simulink model "MobileManipulatorSlave"  (R2016a)
settings: Solver=FixedStepDiscrete  SolverMode=SingleTasking  StartTime=0.0  StopTime=inf  FixedStep=.001  RelTol=1e-3
undefined symbols (not defined in the file): DiscIntNeverNeededParam, transl
libraries: simulink x18, dspfactors x1, LibrarySimulinkSAS x1, aerolibanimutils x1, dspnetwork x1
settings Model: xpc_rtwmakecfg_data=_jpeg_  Creator=DSANTIAGO  LastModifiedBy=INAUT
settings DataIOCC: LimitDataPoints=on  SaveFormat=Array
settings OptimizationCC: BlockReduction=off  BooleanDataType=off
settings DebuggingCC: SaveWithParameterizedLinksMsg=none  UnderspecifiedInitializationDetection=Classic  MergeDetectMultiDrivingBlocksExec=none  SignalResolutionControl=TryResolveAllWithWarning  InvalidFcnCallConnMsg=warning  FcnCallInpInsideContextMsg=EnableAllAsWarning
settings HardwareCC: ProdBitPerPointer=32  ProdLargestAtomicFloat=None  ProdIntDivRoundTo=Undefined  ProdEndianess=Unspecified  ProdWordSize=32  ProdHWDeviceType=32-bit Generic  TargetUnknown=on
settings ModelReferenceCC: PropagateSignalLabelsOutOfModel=off
settings ConfigComp: CovSFcnEnable=off

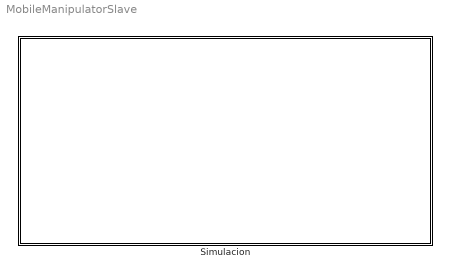
== system MobileManipulatorSlave ==
  Simulacion : Subsystem  mask{sel=1, offSet=[1.5e-1 0 0.1]', h1=.01, h2=.01, kgmb=diag([8 10]), kgms=diag([4 4 4]), kms=10, kmb=5, ksb=1}
      mask prompts: sel "Control (s/m)"; h1 "Delay1"; h2 "Delay2"

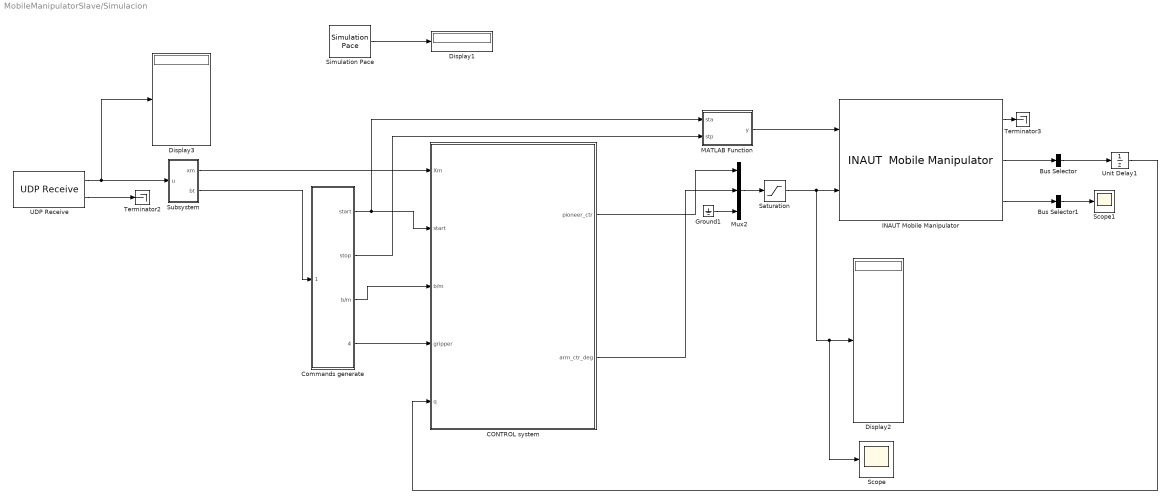
== system MobileManipulatorSlave/Simulacion ==
  Bus Selector : BusSelector  OutputSignals=q_{arm}  OutputAsBus=on
  Bus Selector1 : BusSelector  OutputSignals=base Info.current rigth motor?,base Info.current left motor?  OutputAsBus=on
  CONTROL system : Subsystem
  Commands generate : Subsystem
  Display1 : Display
  Display2 : Display
  Display3 : Display
  Ground1 : Ground
  INAUT Mobile Manipulator : LibrarySimulinkSAS/INAUT  Mobile Manipulator  IdB=3  IdM=1  IdL=0  ts=-1
  MATLAB Function : MATLAB Function  TreatAsAtomicUnit=on
  Mux2 : Mux  Inputs=3
  Saturation : Saturate  UpperLimit=2000  LowerLimit=-2000
  Scope : Scope
  Scope1 : Scope
  Simulation Pace : aerolibanimutils/Simulation Pace  SimulationPace=1  SleepMode=MATLAB Thread  OutputPaceError=on  SampleTime=-1
  Subsystem : Subsystem
  Terminator2 : Terminator
  Terminator3 : Terminator
  UDP Receive : dspnetwork/UDP Receive  localURL='0.0.0.0'  localPort=24102  remoteURL='192.168.1.103'  remotePort=-1  recvBufferSize=1024  dims=7  signalDatatype=double  isVarSize=off  showBlockingTime=off  blockingTime=0  sampletime=-1  blockPlatform=[]
  Unit Delay1 : UnitDelay  SampleTime=-1
  wires:
  Subsystem/1(xm) -> CONTROL system/1(Xm)
  Unit Delay1/1 -> CONTROL system/5(q)
  Subsystem/2(bt) -> Commands generate/1(butons)
  Commands generate/1(start) -> MATLAB Function/1(sta), CONTROL system/2(start)
  CONTROL system/2(arm_ctr_deg) -> Mux2/2
  Mux2/1 -> Saturation/1
  INAUT Mobile Manipulator/2 -> Bus Selector/1
  INAUT Mobile Manipulator/3 -> Bus Selector1/1
  INAUT Mobile Manipulator/1 -> Terminator3/1
  Bus Selector/1 -> Unit Delay1/1
  CONTROL system/1(pioneer_ctr) -> Mux2/1
  Ground1/1 -> Mux2/3
  Simulation Pace/1 -> Display1/1
  Commands generate/3(b/m) -> CONTROL system/3(b/m)
  Commands generate/4(griper) -> CONTROL system/4(gripper)
  UDP Receive/1 -> Subsystem/1(u), Display3/1
  UDP Receive/2 -> Terminator2/1
  Saturation/1 -> Scope/1, Display2/1, INAUT Mobile Manipulator/2
  Bus Selector1/1 -> Scope1/1
  MATLAB Function/1(y) -> INAUT Mobile Manipulator/1
  Commands generate/2(stop) -> MATLAB Function/2(stp)

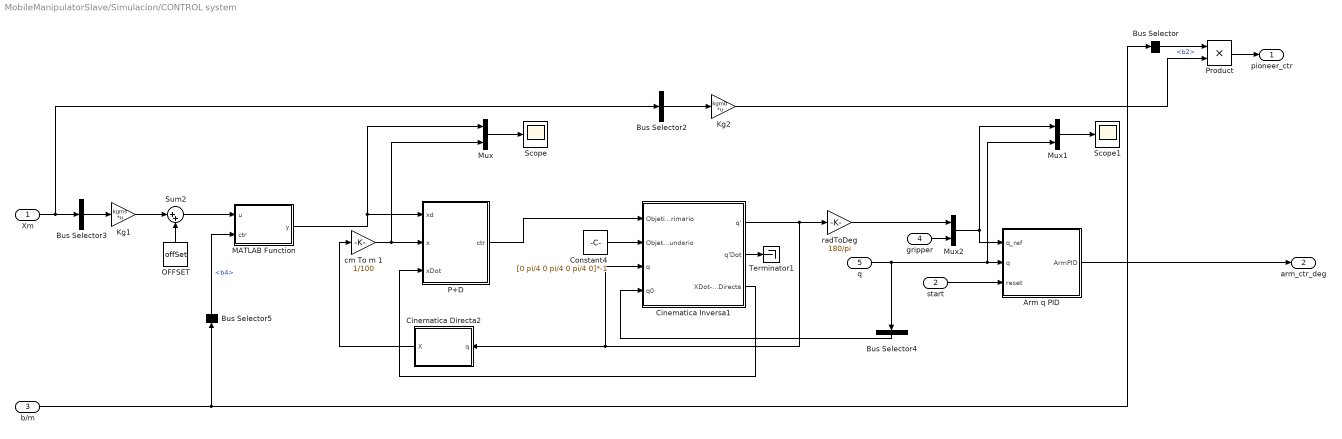
== system MobileManipulatorSlave/Simulacion/CONTROL system ==
  Xm : Inport
  start : Inport  Port=2
  b/m : Inport  Port=3
  gripper : Inport  Port=4
  q : Inport  Port=5
  Arm q PID : Subsystem
  Bus Selector : BusSelector  OutputSignals=b2
  Bus Selector2 : BusSelector  OutputSignals=x,y  OutputAsBus=on
  Bus Selector3 : BusSelector  OutputSignals=x,y,z  OutputAsBus=on
  Bus Selector4 : BusSelector  OutputSignals=q1,q2,q3,q4,q5,q6,q7  OutputAsBus=on
  Bus Selector5 : BusSelector  OutputSignals=b4
  Cinematica Directa2 : Subsystem
  Cinematica Inversa1 : Subsystem
  Constant4 : Constant  Value=[0 pi/4 0 pi/4 0 pi/4 0]*-1
  Kg1 : Gain  Gain=kgms  Multiplication=Matrix(K*u)
  Kg2 : Gain  Gain=kgmb  Multiplication=Matrix(K*u)
  MATLAB Function : MATLAB Function  TreatAsAtomicUnit=on
  Mux : Mux  Inputs=2
  Mux1 : Mux  Inputs=2
  Mux2 : Mux  Inputs=2
  OFFSET : Constant  Value=offSet
  P+D : Subsystem
  Product : Product
  Scope : Scope
  Scope1 : Scope
  Sum2 : Sum  Inputs=|++
  Terminator1 : Terminator
  cm To m 1 : Gain  Gain=1/100
  radToDeg : Gain  Gain=180/pi
  pioneer_ctr : Outport
  arm_ctr_deg : Outport  Port=2
  wires:
  Xm/1 -> Bus Selector3/1, Bus Selector2/1
  Bus Selector2/1 -> Kg2/1
  Cinematica Inversa1/1(q') -> Cinematica Inversa1/3(q), Cinematica Directa2/1(q), radToDeg/1
  OFFSET/1 -> Sum2/2
  Kg1/1 -> Sum2/1
  P+D/1(ctr) -> Cinematica Inversa1/1(Objetivo Primario)
  Cinematica Directa2/1("X ") -> cm To m 1/1
  cm To m 1/1 -> Mux/2, P+D/2(x)
  Constant4/1 -> Cinematica Inversa1/2(Objetivo Secundario)
  gripper/1 -> Mux2/2
  start/1 -> Arm q PID/3(reset)
  b/m/1 -> Bus Selector5/1, Bus Selector/1
  Bus Selector/1 -> Product/1  "<b2>"
  Kg2/1 -> Product/2
  radToDeg/1 -> Mux2/1
  Sum2/1 -> MATLAB Function/1(u)
  Product/1 -> pioneer_ctr/1
  Cinematica Inversa1/2(q'Dot) -> Terminator1/1
  Bus Selector3/1 -> Kg1/1
  Mux/1 -> Scope/1
  Cinematica Inversa1/3(XDot- CinematicaDirecta) -> P+D/3(xDot)
  q/1 -> Bus Selector4/1, Mux1/2, Arm q PID/2(q)
  Mux2/1 -> Mux1/1, Arm q PID/1(q_ref)
  Mux1/1 -> Scope1/1
  Bus Selector4/1 -> Cinematica Inversa1/4(q0)
  MATLAB Function/1(y) -> Mux/1, P+D/1(xd)
  Bus Selector5/1 -> MATLAB Function/2(ctr)  "<b4>"
  Arm q PID/1(ArmPID) -> arm_ctr_deg/1

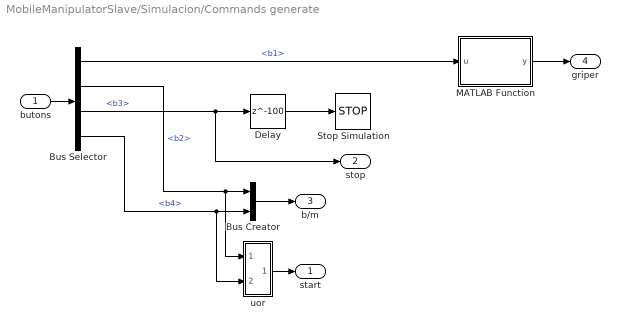
== system MobileManipulatorSlave/Simulacion/Commands generate ==
  butons : Inport
  Bus Creator : BusCreator  Inputs=2
  Bus Selector : BusSelector  OutputSignals=b1,b2,b3,b4
  Delay : Delay  DelayLength=100
  MATLAB Function : MATLAB Function  TreatAsAtomicUnit=on
  Stop Simulation : Stop
  uor : Subsystem
  start : Outport
  stop : Outport  Port=2
  b/m : Outport  Port=3
  griper : Outport  Port=4
  wires:
  Bus Selector/2 -> uor/1(u1), Bus Creator/1  "<b2>"
  Bus Selector/3 -> stop/1, Delay/1  "<b3>"
  Delay/1 -> Stop Simulation/1
  Bus Creator/1 -> b/m/1
  Bus Selector/4 -> uor/2(u2), Bus Creator/2  "<b4>"
  Bus Selector/1 -> MATLAB Function/1(u)  "<b1>"
  butons/1 -> Bus Selector/1
  uor/1(y) -> start/1
  MATLAB Function/1(y) -> griper/1

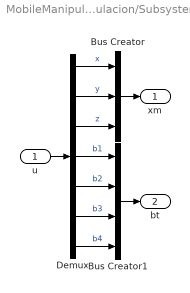
== system MobileManipulatorSlave/Simulacion/Subsystem ==
  u : Inport
  Bus Creator : BusCreator  Inputs=3
  Bus Creator1 : BusCreator  Inputs=4
  Demux : Demux  Outputs=7
  xm : Outport
  bt : Outport  Port=2
  wires:
  Demux/2 -> Bus Creator/2  "y"
  Demux/3 -> Bus Creator/3  "z"
  Demux/5 -> Bus Creator1/2  "b2"
  Demux/1 -> Bus Creator/1  "x"
  Demux/6 -> Bus Creator1/3  "b3"
  Demux/4 -> Bus Creator1/1  "b1"
  Demux/7 -> Bus Creator1/4  "b4"
  Bus Creator1/1 -> bt/1
  u/1 -> Demux/1
  Bus Creator/1 -> xm/1

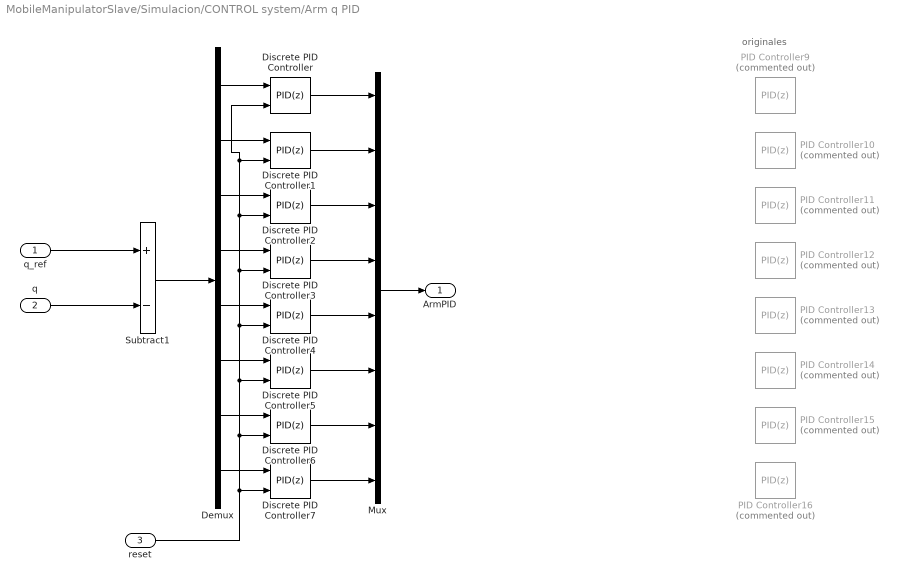
== system MobileManipulatorSlave/Simulacion/CONTROL system/Arm q PID ==
  note: originales
  q_ref : Inport
  q : Inport  Port=2
  reset : Inport  Port=3
  Demux : Demux  Outputs=8
  Discrete PID Controller : simulink/Continuous/PID Controller  Controller=PID  TimeDomain=Discrete-time  SampleTime=-1  IntegratorMethod=Forward Euler  FilterMethod=Forward Euler  Form=Parallel  UseFilter=on  ControllerParametersSource=internal  P=125  I=40  D=0.01  N=100  InitialConditionSource=internal  InitialConditionForIntegrator=0  InitialConditionForFilter=0  ExternalReset=level  LimitOutput=on  UpperSaturationLimit=4095  LowerSaturationLimit=-4095  LinearizeAsGain=on  AntiWindupMode=clamping  Kb=1  TrackingMode=off  Kt=1  PParamMin=[]  PParamMax=[]  IParamMin=[]  IParamMax=[]  DParamMin=[]  DParamMax=[]  NParamMin=[]  NParamMax=[]  KbParamMin=[]  KbParamMax=[]  KtParamMin=[]  KtParamMax=[]  POutMin=[]  POutMax=[]  IOutMin=[]  IOutMax=[]  DOutMin=[]  DOutMax=[]  NOutMin=[]  NOutMax=[]  KbOutMin=[]  KbOutMax=[]  KtOutMin=[]  KtOutMax=[]  IntegratorOutMin=[]  IntegratorOutMax=[]  FilterOutMin=[]  FilterOutMax=[]  SumOutMin=[]  SumOutMax=[]  SumI1OutMin=[]  SumI1OutMax=[]  SumI2OutMin=[]  SumI2OutMax=[]  SumI3OutMin=[]  SumI3OutMax=[]  SumDOutMin=[]  SumDOutMax=[]  SaturationOutMin=[]  SaturationOutMax=[]  IntegratorContinuousStateAttributes=''  IntegratorStateMustResolveToSignalObject=off  IntegratorRTWStateStorageClass=Auto  FilterContinuousStateAttributes=''  FilterStateMustResolveToSignalObject=off  FilterRTWStateStorageClass=Auto  DifferentiatorICPrevScaledInput=0  DifferentiatorOutMin=[]  DifferentiatorOutMax=[]
  Discrete PID Controller1 : simulink/Continuous/PID Controller  Controller=PID  TimeDomain=Discrete-time  SampleTime=-1  IntegratorMethod=Forward Euler  FilterMethod=Forward Euler  Form=Parallel  UseFilter=on  ControllerParametersSource=internal  P=75  I=100  D=0.01  N=100  InitialConditionSource=internal  InitialConditionForIntegrator=0  InitialConditionForFilter=0  ExternalReset=level  LimitOutput=on  UpperSaturationLimit=4095  LowerSaturationLimit=-4095  LinearizeAsGain=on  AntiWindupMode=clamping  Kb=1  TrackingMode=off  Kt=1  PParamMin=[]  PParamMax=[]  IParamMin=[]  IParamMax=[]  DParamMin=[]  DParamMax=[]  NParamMin=[]  NParamMax=[]  KbParamMin=[]  KbParamMax=[]  KtParamMin=[]  KtParamMax=[]  POutMin=[]  POutMax=[]  IOutMin=[]  IOutMax=[]  DOutMin=[]  DOutMax=[]  NOutMin=[]  NOutMax=[]  KbOutMin=[]  KbOutMax=[]  KtOutMin=[]  KtOutMax=[]  IntegratorOutMin=[]  IntegratorOutMax=[]  FilterOutMin=[]  FilterOutMax=[]  SumOutMin=[]  SumOutMax=[]  SumI1OutMin=[]  SumI1OutMax=[]  SumI2OutMin=[]  SumI2OutMax=[]  SumI3OutMin=[]  SumI3OutMax=[]  SumDOutMin=[]  SumDOutMax=[]  SaturationOutMin=[]  SaturationOutMax=[]  IntegratorContinuousStateAttributes=''  IntegratorStateMustResolveToSignalObject=off  IntegratorRTWStateStorageClass=Auto  FilterContinuousStateAttributes=''  FilterStateMustResolveToSignalObject=off  FilterRTWStateStorageClass=Auto  DifferentiatorICPrevScaledInput=0  DifferentiatorOutMin=[]  DifferentiatorOutMax=[]
  Discrete PID Controller2 : simulink/Continuous/PID Controller  Controller=PID  TimeDomain=Discrete-time  SampleTime=-1  IntegratorMethod=Forward Euler  FilterMethod=Forward Euler  Form=Parallel  UseFilter=on  ControllerParametersSource=internal  P=80  I=45  D=0.01  N=100  InitialConditionSource=internal  InitialConditionForIntegrator=0  InitialConditionForFilter=0  ExternalReset=level  LimitOutput=on  UpperSaturationLimit=4095  LowerSaturationLimit=-4095  LinearizeAsGain=on  AntiWindupMode=clamping  Kb=1  TrackingMode=off  Kt=1  PParamMin=[]  PParamMax=[]  IParamMin=[]  IParamMax=[]  DParamMin=[]  DParamMax=[]  NParamMin=[]  NParamMax=[]  KbParamMin=[]  KbParamMax=[]  KtParamMin=[]  KtParamMax=[]  POutMin=[]  POutMax=[]  IOutMin=[]  IOutMax=[]  DOutMin=[]  DOutMax=[]  NOutMin=[]  NOutMax=[]  KbOutMin=[]  KbOutMax=[]  KtOutMin=[]  KtOutMax=[]  IntegratorOutMin=[]  IntegratorOutMax=[]  FilterOutMin=[]  FilterOutMax=[]  SumOutMin=[]  SumOutMax=[]  SumI1OutMin=[]  SumI1OutMax=[]  SumI2OutMin=[]  SumI2OutMax=[]  SumI3OutMin=[]  SumI3OutMax=[]  SumDOutMin=[]  SumDOutMax=[]  SaturationOutMin=[]  SaturationOutMax=[]  IntegratorContinuousStateAttributes=''  IntegratorStateMustResolveToSignalObject=off  IntegratorRTWStateStorageClass=Auto  FilterContinuousStateAttributes=''  FilterStateMustResolveToSignalObject=off  FilterRTWStateStorageClass=Auto  DifferentiatorICPrevScaledInput=0  DifferentiatorOutMin=[]  DifferentiatorOutMax=[]
  Discrete PID Controller{3..7} (5 alike) : simulink/Continuous/PID Controller  Controller=PID  TimeDomain=Discrete-time  SampleTime=-1  IntegratorMethod=Forward Euler  FilterMethod=Forward Euler  Form=Parallel  UseFilter=on  ControllerParametersSource=internal  P=75  I=40  D=0.01  N=100  InitialConditionSource=internal  InitialConditionForIntegrator=0  InitialConditionForFilter=0  ExternalReset=level  LimitOutput=on  UpperSaturationLimit=4095  LowerSaturationLimit=-4095  LinearizeAsGain=on  AntiWindupMode=clamping  Kb=1  TrackingMode=off  Kt=1  PParamMin=[]  PParamMax=[]  IParamMin=[]  IParamMax=[]  DParamMin=[]  DParamMax=[]  NParamMin=[]  NParamMax=[]  KbParamMin=[]  KbParamMax=[]  KtParamMin=[]  KtParamMax=[]  POutMin=[]  POutMax=[]  IOutMin=[]  IOutMax=[]  DOutMin=[]  DOutMax=[]  NOutMin=[]  NOutMax=[]  KbOutMin=[]  KbOutMax=[]  KtOutMin=[]  KtOutMax=[]  IntegratorOutMin=[]  IntegratorOutMax=[]  FilterOutMin=[]  FilterOutMax=[]  SumOutMin=[]  SumOutMax=[]  SumI1OutMin=[]  SumI1OutMax=[]  SumI2OutMin=[]  SumI2OutMax=[]  SumI3OutMin=[]  SumI3OutMax=[]  SumDOutMin=[]  SumDOutMax=[]  SaturationOutMin=[]  SaturationOutMax=[]  IntegratorContinuousStateAttributes=''  IntegratorStateMustResolveToSignalObject=off  IntegratorRTWStateStorageClass=Auto  FilterContinuousStateAttributes=''  FilterStateMustResolveToSignalObject=off  FilterRTWStateStorageClass=Auto  DifferentiatorICPrevScaledInput=0  DifferentiatorOutMin=[]  DifferentiatorOutMax=[]
  Mux : Mux  Inputs=8
  PID Controller10 : simulink/Continuous/PID Controller  Commented=on  Controller=PID  TimeDomain=Discrete-time  SampleTime=-1  IntegratorMethod=Forward Euler  FilterMethod=Forward Euler  Form=Parallel  UseFilter=on  ControllerParametersSource=internal  P=75  I=100  D=0.01  N=100  InitialConditionSource=internal  InitialConditionForIntegrator=0  InitialConditionForFilter=0  ExternalReset=rising  LimitOutput=on  UpperSaturationLimit=4095  LowerSaturationLimit=-4095  LinearizeAsGain=on  AntiWindupMode=clamping  Kb=1  TrackingMode=off  Kt=1  PParamMin=[]  PParamMax=[]  PParamDataTypeStr=single  IParamMin=[]  IParamMax=[]  IParamDataTypeStr=single  DParamMin=[]  DParamMax=[]  DParamDataTypeStr=single  NParamMin=[]  NParamMax=[]  NParamDataTypeStr=single  KbParamMin=[]  KbParamMax=[]  KtParamMin=[]  KtParamMax=[]  POutMin=[]  POutMax=[]  POutDataTypeStr=single  PGainOutDataTypeStr=single  PProdOutDataTypeStr=single  IOutMin=[]  IOutMax=[]  IOutDataTypeStr=single  IGainOutDataTypeStr=single  IProdOutDataTypeStr=single  DOutMin=[]  DOutMax=[]  DOutDataTypeStr=single  DGainOutDataTypeStr=single  DProdOutDataTypeStr=single  NOutMin=[]  NOutMax=[]  NOutDataTypeStr=single  NGainOutDataTypeStr=single  NProdOutDataTypeStr=single  KbOutMin=[]  KbOutMax=[]  KtOutMin=[]  KtOutMax=[]  IntegratorOutMin=[]  IntegratorOutMax=[]  IntegratorOutDataTypeStr=single  FilterOutMin=[]  FilterOutMax=[]  FilterOutDataTypeStr=single  SumOutMin=[]  SumOutMax=[]  SumOutDataTypeStr=single  SumI1OutMin=[]  SumI1OutMax=[]  SumI2OutMin=[]  SumI2OutMax=[]  SumI3OutMin=[]  SumI3OutMax=[]  SumDOutMin=[]  SumDOutMax=[]  SumDOutDataTypeStr=single  SumAccumDataTypeStr=single  SumDAccumDataTypeStr=single  SaturationOutMin=[]  SaturationOutMax=[]  SaturationOutDataTypeStr=single  IntegratorContinuousStateAttributes=''  IntegratorStateMustResolveToSignalObject=off  IntegratorRTWStateStorageClass=Auto  FilterContinuousStateAttributes=''  FilterStateMustResolveToSignalObject=off  FilterRTWStateStorageClass=Auto  DifferentiatorICPrevScaledInput=0  DifferentiatorOutMin=[]  DifferentiatorOutMax=[]
  PID Controller11 : simulink/Continuous/PID Controller  Commented=on  Controller=PID  TimeDomain=Discrete-time  SampleTime=-1  IntegratorMethod=Forward Euler  FilterMethod=Forward Euler  Form=Parallel  UseFilter=on  ControllerParametersSource=internal  P=80  I=45  D=0.01  N=100  InitialConditionSource=internal  InitialConditionForIntegrator=0  InitialConditionForFilter=0  ExternalReset=rising  LimitOutput=on  UpperSaturationLimit=4095  LowerSaturationLimit=-4095  LinearizeAsGain=on  AntiWindupMode=clamping  Kb=1  TrackingMode=off  Kt=1  PParamMin=[]  PParamMax=[]  PParamDataTypeStr=single  IParamMin=[]  IParamMax=[]  IParamDataTypeStr=single  DParamMin=[]  DParamMax=[]  DParamDataTypeStr=single  NParamMin=[]  NParamMax=[]  NParamDataTypeStr=single  KbParamMin=[]  KbParamMax=[]  KtParamMin=[]  KtParamMax=[]  POutMin=[]  POutMax=[]  POutDataTypeStr=single  PGainOutDataTypeStr=single  PProdOutDataTypeStr=single  IOutMin=[]  IOutMax=[]  IOutDataTypeStr=single  IGainOutDataTypeStr=single  IProdOutDataTypeStr=single  DOutMin=[]  DOutMax=[]  DOutDataTypeStr=single  DGainOutDataTypeStr=single  DProdOutDataTypeStr=single  NOutMin=[]  NOutMax=[]  NOutDataTypeStr=single  NGainOutDataTypeStr=single  NProdOutDataTypeStr=single  KbOutMin=[]  KbOutMax=[]  KtOutMin=[]  KtOutMax=[]  IntegratorOutMin=[]  IntegratorOutMax=[]  IntegratorOutDataTypeStr=single  FilterOutMin=[]  FilterOutMax=[]  FilterOutDataTypeStr=single  SumOutMin=[]  SumOutMax=[]  SumOutDataTypeStr=single  SumI1OutMin=[]  SumI1OutMax=[]  SumI2OutMin=[]  SumI2OutMax=[]  SumI3OutMin=[]  SumI3OutMax=[]  SumDOutMin=[]  SumDOutMax=[]  SumDOutDataTypeStr=single  SumAccumDataTypeStr=single  SumDAccumDataTypeStr=single  SaturationOutMin=[]  SaturationOutMax=[]  SaturationOutDataTypeStr=single  IntegratorContinuousStateAttributes=''  IntegratorStateMustResolveToSignalObject=off  IntegratorRTWStateStorageClass=Auto  FilterContinuousStateAttributes=''  FilterStateMustResolveToSignalObject=off  FilterRTWStateStorageClass=Auto  DifferentiatorICPrevScaledInput=0  DifferentiatorOutMin=[]  DifferentiatorOutMax=[]
  PID Controller{12..16} (5 alike) : simulink/Continuous/PID Controller  Commented=on  Controller=PID  TimeDomain=Discrete-time  SampleTime=-1  IntegratorMethod=Forward Euler  FilterMethod=Forward Euler  Form=Parallel  UseFilter=on  ControllerParametersSource=internal  P=75  I=40  D=0.01  N=100  InitialConditionSource=internal  InitialConditionForIntegrator=0  InitialConditionForFilter=0  ExternalReset=rising  LimitOutput=on  UpperSaturationLimit=4095  LowerSaturationLimit=-4095  LinearizeAsGain=on  AntiWindupMode=clamping  Kb=1  TrackingMode=off  Kt=1  PParamMin=[]  PParamMax=[]  PParamDataTypeStr=single  IParamMin=[]  IParamMax=[]  IParamDataTypeStr=single  DParamMin=[]  DParamMax=[]  DParamDataTypeStr=single  NParamMin=[]  NParamMax=[]  NParamDataTypeStr=single  KbParamMin=[]  KbParamMax=[]  KtParamMin=[]  KtParamMax=[]  POutMin=[]  POutMax=[]  POutDataTypeStr=single  PGainOutDataTypeStr=single  PProdOutDataTypeStr=single  IOutMin=[]  IOutMax=[]  IOutDataTypeStr=single  IGainOutDataTypeStr=single  IProdOutDataTypeStr=single  DOutMin=[]  DOutMax=[]  DOutDataTypeStr=single  DGainOutDataTypeStr=single  DProdOutDataTypeStr=single  NOutMin=[]  NOutMax=[]  NOutDataTypeStr=single  NGainOutDataTypeStr=single  NProdOutDataTypeStr=single  KbOutMin=[]  KbOutMax=[]  KtOutMin=[]  KtOutMax=[]  IntegratorOutMin=[]  IntegratorOutMax=[]  IntegratorOutDataTypeStr=single  FilterOutMin=[]  FilterOutMax=[]  FilterOutDataTypeStr=single  SumOutMin=[]  SumOutMax=[]  SumOutDataTypeStr=single  SumI1OutMin=[]  SumI1OutMax=[]  SumI2OutMin=[]  SumI2OutMax=[]  SumI3OutMin=[]  SumI3OutMax=[]  SumDOutMin=[]  SumDOutMax=[]  SumDOutDataTypeStr=single  SumAccumDataTypeStr=single  SumDAccumDataTypeStr=single  SaturationOutMin=[]  SaturationOutMax=[]  SaturationOutDataTypeStr=single  IntegratorContinuousStateAttributes=''  IntegratorStateMustResolveToSignalObject=off  IntegratorRTWStateStorageClass=Auto  FilterContinuousStateAttributes=''  FilterStateMustResolveToSignalObject=off  FilterRTWStateStorageClass=Auto  DifferentiatorICPrevScaledInput=0  DifferentiatorOutMin=[]  DifferentiatorOutMax=[]
  PID Controller9 : simulink/Continuous/PID Controller  Commented=on  Controller=PID  TimeDomain=Discrete-time  SampleTime=-1  IntegratorMethod=Forward Euler  FilterMethod=Forward Euler  Form=Parallel  UseFilter=on  ControllerParametersSource=internal  P=125  I=40  D=0.01  N=100  InitialConditionSource=internal  InitialConditionForIntegrator=0  InitialConditionForFilter=0  ExternalReset=level  LimitOutput=on  UpperSaturationLimit=4095  LowerSaturationLimit=-4095  LinearizeAsGain=on  AntiWindupMode=clamping  Kb=1  TrackingMode=off  Kt=1  PParamMin=[]  PParamMax=[]  PParamDataTypeStr=single  IParamMin=[]  IParamMax=[]  IParamDataTypeStr=single  DParamMin=[]  DParamMax=[]  DParamDataTypeStr=single  NParamMin=[]  NParamMax=[]  NParamDataTypeStr=single  KbParamMin=[]  KbParamMax=[]  KtParamMin=[]  KtParamMax=[]  POutMin=[]  POutMax=[]  POutDataTypeStr=single  PGainOutDataTypeStr=single  PProdOutDataTypeStr=single  IOutMin=[]  IOutMax=[]  IOutDataTypeStr=single  IGainOutDataTypeStr=single  IProdOutDataTypeStr=single  DOutMin=[]  DOutMax=[]  DOutDataTypeStr=single  DGainOutDataTypeStr=single  DProdOutDataTypeStr=single  NOutMin=[]  NOutMax=[]  NOutDataTypeStr=single  NGainOutDataTypeStr=single  NProdOutDataTypeStr=single  KbOutMin=[]  KbOutMax=[]  KtOutMin=[]  KtOutMax=[]  IntegratorOutMin=[]  IntegratorOutMax=[]  IntegratorOutDataTypeStr=single  FilterOutMin=[]  FilterOutMax=[]  FilterOutDataTypeStr=single  SumOutMin=[]  SumOutMax=[]  SumOutDataTypeStr=single  SumI1OutMin=[]  SumI1OutMax=[]  SumI2OutMin=[]  SumI2OutMax=[]  SumI3OutMin=[]  SumI3OutMax=[]  SumDOutMin=[]  SumDOutMax=[]  SumDOutDataTypeStr=single  SumAccumDataTypeStr=single  SumDAccumDataTypeStr=single  SaturationOutMin=[]  SaturationOutMax=[]  SaturationOutDataTypeStr=single  IntegratorContinuousStateAttributes=''  IntegratorStateMustResolveToSignalObject=off  IntegratorRTWStateStorageClass=Auto  FilterContinuousStateAttributes=''  FilterStateMustResolveToSignalObject=off  FilterRTWStateStorageClass=Auto  DifferentiatorICPrevScaledInput=0  DifferentiatorOutMin=[]  DifferentiatorOutMax=[]
  Subtract1 : Sum  Inputs=+-
  ArmPID : Outport  PortDimensions=8
  wires:
  q/1 -> Subtract1/2
  q_ref/1 -> Subtract1/1
  Demux/1 -> Discrete PID Controller/1
  Subtract1/1 -> Demux/1
  Demux/6 -> Discrete PID Controller5/1
  Demux/2 -> Discrete PID Controller1/1
  Demux/3 -> Discrete PID Controller2/1
  Demux/4 -> Discrete PID Controller3/1
  Demux/5 -> Discrete PID Controller4/1
  Demux/7 -> Discrete PID Controller6/1
  Demux/8 -> Discrete PID Controller7/1
  Discrete PID Controller7/1 -> Mux/8
  Discrete PID Controller6/1 -> Mux/7
  Discrete PID Controller5/1 -> Mux/6
  Discrete PID Controller4/1 -> Mux/5
  Discrete PID Controller3/1 -> Mux/4
  Discrete PID Controller2/1 -> Mux/3
  Discrete PID Controller1/1 -> Mux/2
  reset/1 -> Discrete PID Controller7/2, Discrete PID Controller6/2, Discrete PID Controller5/2, Discrete PID Controller4/2, Discrete PID Controller3/2, Discrete PID Controller2/2, Discrete PID Controller1/2, Discrete PID Controller/2
  Discrete PID Controller/1 -> Mux/1
  Mux/1 -> ArmPID/1

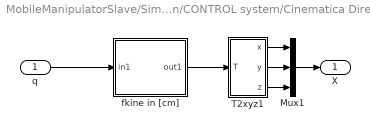
== system MobileManipulatorSlave/Simulacion/CONTROL system/Cinematica Directa2 ==
  q : Inport
  Mux1 : Mux  Inputs=3
  T2xyz1 : Subsystem
      mask help: Convert transform to xyz scalars
      mask Help:
      | Convert homogeneous transformation to position scalars.
      | 
      | 
      | <b>Inputs::</b>
      | 
      | T (4x4) a translation represented as a homogeneous transformation
      | 
      | <b>Outputs::</b>
      | 
      | x (1x1) x-coordinate
      | y (1x1) y-coordinate
      | z (1x1) z-coordinate
      | 
      | <b>Notes::</b>
      | 
      | - A wrapper for the Toolbox function transl().
  fkine in [cm] : MATLAB Function  TreatAsAtomicUnit=on
  "X " : Outport
  wires:
  fkine in [cm]/1(out1) -> T2xyz1/1(T)
  Mux1/1 -> "X "/1
  T2xyz1/1(x) -> Mux1/1
  T2xyz1/2(y) -> Mux1/2
  T2xyz1/3(z) -> Mux1/3
  q/1 -> fkine in [cm]/1(in1)

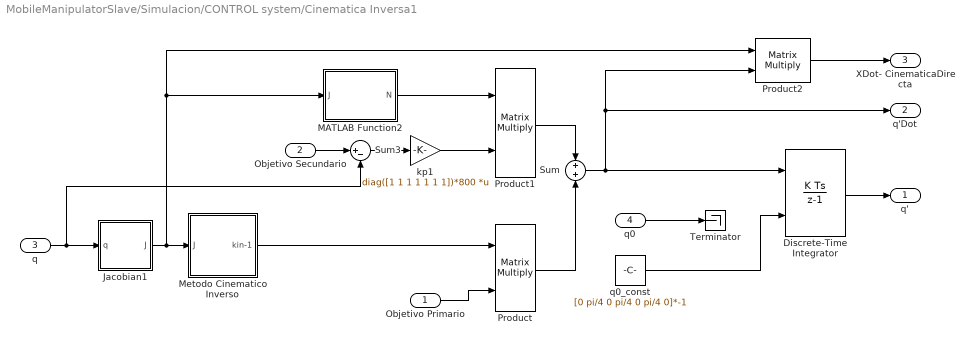
== system MobileManipulatorSlave/Simulacion/CONTROL system/Cinematica Inversa1 ==
  Objetivo Primario : Inport
  Objetivo Secundario : Inport  Port=2
  q : Inport  Port=3
  q0 : Inport  Port=4
  Discrete-Time Integrator : DiscreteIntegrator  InitialConditionSource=external  InitialConditionSetting=State (most efficient)  SampleTime=-1  ICPrevOutput=DiscIntNeverNeededParam  ICPrevScaledInput=DiscIntNeverNeededParam
  Jacobian1 : Subsystem
  MATLAB Function2 : MATLAB Function  TreatAsAtomicUnit=on
  Metodo Cinematico Inverso : Subsystem
  Product : Product  Multiplication=Matrix(*)
  Product1 : Product  Multiplication=Matrix(*)
  Product2 : Product  Multiplication=Matrix(*)
  Sum : Sum
  Sum3 : Sum  Inputs=|+-
  Terminator : Terminator
  kp1 : Gain  Gain=diag([1 1 1 1 1 1 1])*800  Multiplication=Matrix(K*u)
  q0_const : Constant  Value=[0 pi/4 0 pi/4 0 pi/4 0]*-1
  q' : Outport
  q'Dot : Outport  Port=2
  XDot- CinematicaDirecta : Outport  Port=3
  wires:
  MATLAB Function2/1(N) -> Product1/1
  Product1/1 -> Sum/1
  Sum/1 -> Discrete-Time Integrator/1, Product2/2, q'Dot/1
  Product/1 -> Sum/2
  q/1 -> Sum3/2, Jacobian1/1(q)
  Jacobian1/1(J) -> MATLAB Function2/1(J), Product2/1, Metodo Cinematico Inverso/1(J)
  Objetivo Secundario/1 -> Sum3/1
  Sum3/1 -> kp1/1
  kp1/1 -> Product1/2
  Discrete-Time Integrator/1 -> q'/1
  Metodo Cinematico Inverso/1(kin-1) -> Product/1
  Objetivo Primario/1 -> Product/2
  Product2/1 -> XDot- CinematicaDirecta/1
  q0/1 -> Terminator/1
  q0_const/1 -> Discrete-Time Integrator/2

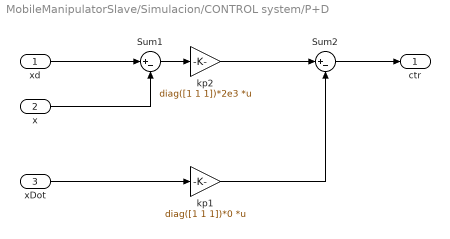
== system MobileManipulatorSlave/Simulacion/CONTROL system/P+D ==
  xd : Inport
  x : Inport  Port=2
  xDot : Inport  Port=3
  Sum1 : Sum  Inputs=|+-
  Sum2 : Sum  Inputs=|+-
  kp1 : Gain  Gain=diag([1 1 1])*0  Multiplication=Matrix(K*u)
  kp2 : Gain  Gain=diag([1 1 1])*2e3  Multiplication=Matrix(K*u)
  ctr : Outport
  wires:
  x/1 -> Sum1/2
  xd/1 -> Sum1/1
  Sum2/1 -> ctr/1
  Sum1/1 -> kp2/1
  xDot/1 -> kp1/1
  kp2/1 -> Sum2/1
  kp1/1 -> Sum2/2

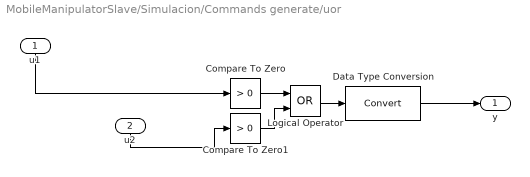
== system MobileManipulatorSlave/Simulacion/Commands generate/uor ==
  u1 : Inport
  u2 : Inport  Port=2
  Compare To Zero : simulink/Logic and Bit Operations/Compare To Zero  relop=>  OutDataTypeStr=boolean
  Compare To Zero1 : simulink/Logic and Bit Operations/Compare To Zero  relop=>  OutDataTypeStr=boolean
  Data Type Conversion : DataTypeConversion
  Logical Operator : Logic  Operator=OR  AllPortsSameDT=off  OutDataTypeStr=boolean
  y : Outport
  wires:
  u2/1 -> Compare To Zero1/1
  Compare To Zero1/1 -> Logical Operator/2
  u1/1 -> Compare To Zero/1
  Compare To Zero/1 -> Logical Operator/1
  Logical Operator/1 -> Data Type Conversion/1
  Data Type Conversion/1 -> y/1

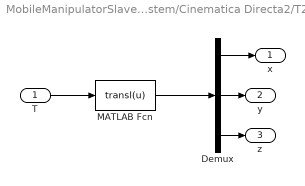
== system MobileManipulatorSlave/Simulacion/CONTROL system/Cinematica Directa2/T2xyz1 ==
  T : Inport
  Demux : Demux  Outputs=3
  MATLAB Fcn : MATLABFcn  MATLABFcn=transl(u)  OutputDimensions=3
  x : Outport
  y : Outport  Port=2
  z : Outport  Port=3
  wires:
  T/1 -> MATLAB Fcn/1
  MATLAB Fcn/1 -> Demux/1
  Demux/1 -> x/1
  Demux/2 -> y/1
  Demux/3 -> z/1

== system MobileManipulatorSlave/Simulacion/CONTROL system/Cinematica Inversa1/Jacobian1 ==
  q : Inport
  MATLAB Function3 : MATLAB Function  TreatAsAtomicUnit=on
  Reshape : Reshape  OutputDimensionality=Row vector (2-D)
  jacob0 : MATLAB Function  TreatAsAtomicUnit=on
  J : Outport
  wires:
  MATLAB Function3/1(J) -> J/1
  q/1 -> Reshape/1
  Reshape/1 -> jacob0/1(in1)
  jacob0/1(out1) -> MATLAB Function3/1(Jc)

== system MobileManipulatorSlave/Simulacion/CONTROL system/Cinematica Inversa1/Metodo Cinematico Inverso ==
  J : Inport
  Inversa sin singularidad : Subsystem
  kin-1 : Outport
  wires:
  J/1 -> Inversa sin singularidad/1(J)
  Inversa sin singularidad/1(invJ) -> kin-1/1

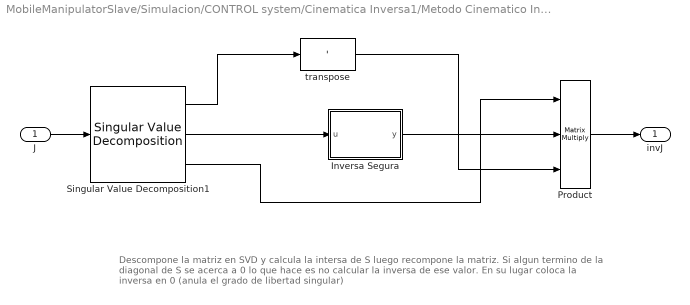
== system MobileManipulatorSlave/Simulacion/CONTROL system/Cinematica Inversa1/Metodo Cinematico Inverso/Inversa sin singularidad ==
  note: Descompone la matriz en SVD y calcula la intersa de S luego recompone la matriz.
      | Si algun termino de la diagonal de S se acerca a 0 lo que hace es no calcular la inversa de ese valor.
      | En su lugar coloca la inversa en 0 (anula el grado de libertad singular)
  J : Inport
  Inversa Segura : MATLAB Function  TreatAsAtomicUnit=on
  Product : Product  Inputs=3  Multiplication=Matrix(*)
  Singular Value Decomposition1 : dspfactors/Singular Value Decomposition  wantv=on  wanterr=off
  transpose : MATLABFcn  MATLABFcn='  Output1D=off
  invJ : Outport
  wires:
  J/1 -> Singular Value Decomposition1/1
  Singular Value Decomposition1/2 -> Inversa Segura/1(u)
  Inversa Segura/1(y) -> Product/2
  Singular Value Decomposition1/1 -> transpose/1
  Product/1 -> invJ/1
  Singular Value Decomposition1/3 -> Product/1
  transpose/1 -> Product/3

== matlab function MobileManipulatorSlave/Simulacion/MATLAB Function ==
  data: sta input; y output; stp input
function y = fcn(sta,stp)
on=[1 1 1];
off=[0 0 0];

if(stp>0)
    y=off;
else
    y=on;
end

== matlab function MobileManipulatorSlave/Simulacion/CONTROL system/MATLAB Function ==
  data: u input; y output; ctr input
function y = fcn(u,ctr)
v=[.39 0 .113]';
if(ctr>0)
    y = u;
else
    y=v;
end

== matlab function MobileManipulatorSlave/Simulacion/Commands generate/MATLAB Function ==
  data: u input; y output
function y = fcn(u)
if u 
    y=-150;
else
    y=100;
end

== matlab function MobileManipulatorSlave/Simulacion/CONTROL system/Cinematica Directa2/fkine in [cm] ==
  data: in1 input; out1 output
function out1 = fkine(in1)
%#codegen

%    This function was generated by the Symbolic Math Toolbox version 6.1.
%    17-Aug-2017 11:24:58

q1 = in1(1,:);
q2 = in1(2,:);
q3 = in1(3,:);
q4 = in1(4,:);
q5 = in1(5,:);
q6 = in1(6,:);
q7 = in1(7,:);
t2 = cos(q1);
t3 = pi.*(1.0./2.0);
t4 = q6+t3;
t5 = cos(q4);
t6 = sin(q1);
t7 = sin(q3);
t8 = t6.*t7;
t9 = cos(q2);
t10 = cos(q3);
t15 = t2.*t9.*t10;
t11 = t8-t15;
t12 = sin(q2);
t13 = sin(q4);
t14 = sin(q5);
t16 = t5.*t11;
t17 = t2.*t12.*t13;
t18 = t16+t17;
t19 = cos(q5);
t20 = t6.*t10;
t21 = t2.*t7.*t9;
t22 = t20+t21;
t23 = sin(q7);
t24 = sin(t4);
t25 = t11.*t13;
t35 = t2.*t5.*t12;
t26 = t25-t35;
t27 = cos(t4);
t28 = t18.*t19;
t29 = t14.*t22;
t30 = t28+t29;
t36 = t24.*t26;
t37 = t27.*t30;
t31 = t36-t37;
t32 = cos(q7);
t33 = t14.*t18;
t38 = t19.*t22;
t34 = t33-t38;
t39 = t2.*t7;
t40 = t6.*t9.*t10;
t41 = t39+t40;
t42 = t5.*t41;
t46 = t6.*t12.*t13;
t43 = t42-t46;
t44 = t2.*t10;
t48 = t6.*t7.*t9;
t45 = t44-t48;
t47 = t14.*t43;
t59 = t19.*t45;
t49 = t47-t59;
t50 = t13.*t41;
t51 = t5.*t6.*t12;
t52 = t50+t51;
t53 = t24.*t52;
t54 = t19.*t43;
t55 = t14.*t45;
t56 = t54+t55;
t58 = t27.*t56;
t57 = t53-t58;
t60 = t9.*t13;
t61 = t5.*t10.*t12;
t62 = t60+t61;
t63 = t14.*t62;
t64 = t7.*t12.*t19;
t65 = t63+t64;
t66 = t19.*t62;
t73 = t7.*t12.*t14;
t67 = t66-t73;
t68 = t27.*t67;
t69 = t5.*t9;
t74 = t10.*t12.*t13;
t70 = t69-t74;
t71 = t24.*t70;
t72 = t68+t71;
out1 = reshape([-t23.*t34+t31.*t32,t23.*t49-t32.*t57,t23.*t65+t32.*t72,0.0,-t23.*t31-t32.*t34,t23.*t57+t32.*t49,-t23.*t72+t32.*t65,0.0,-t26.*t27-t24.*t30,t27.*t52+t24.*t56,cos(q6).*(-t73+t9.*t13.*t19+t5.*t10.*t12.*t19)+t70.*sin(q6),0.0,t2.*t12.*-1.5e1+t11.*t13.*1.7e1+t24.*t26.*8.0-t23.*t34.*8.0-t27.*t30.*8.0+t31.*t32.*8.0-t2.*t5.*t12.*1.7e1,t6.*t12.*-1.5e1-t13.*t41.*1.7e1+t23.*t49.*8.0-t24.*t52.*8.0+t27.*t56.*8.0-t32.*t57.*8.0-t5.*t6.*t12.*1.7e1,t9.*1.5e1+t5.*t9.*1.7e1+t23.*t65.*8.0+t24.*t70.*8.0+t27.*t67.*8.0+t32.*t72.*8.0-t10.*t12.*t13.*1.7e1+1.2e1,1.0],[4, 4]);

== matlab function MobileManipulatorSlave/Simulacion/CONTROL system/Cinematica Inversa1/Jacobian1/MATLAB Function3 ==
  data: Jc input; J output
function J = Jaco(Jc)
J = Jc(1:3,:);

== matlab function MobileManipulatorSlave/Simulacion/CONTROL system/Cinematica Inversa1/Jacobian1/jacob0 ==
  data: in1 input; out1 output
function out1 = jacob0(in1)
%#codegen

%    This function was generated by the Symbolic Math Toolbox version 6.1.
%    17-Aug-2017 11:26:19

q1 = in1(:,1);
q2 = in1(:,2);
q3 = in1(:,3);
q4 = in1(:,4);
q5 = in1(:,5);
q6 = in1(:,6);
q7 = in1(:,7);
t2 = cos(q1);
t3 = pi.*(1.0./2.0);
t4 = q6+t3;
t5 = cos(q4);
t6 = sin(q1);
t7 = sin(q3);
t8 = t6.*t7;
t9 = cos(q2);
t10 = cos(q3);
t15 = t2.*t9.*t10;
t11 = t8-t15;
t12 = sin(q2);
t13 = sin(q4);
t14 = sin(q5);
t16 = t5.*t11;
t17 = t2.*t12.*t13;
t18 = t16+t17;
t19 = cos(q5);
t20 = t6.*t10;
t21 = t2.*t7.*t9;
t22 = t20+t21;
t23 = cos(q7);
t24 = sin(q6);
t25 = cos(q6);
t26 = sin(q7);
t27 = cos(t4);
t28 = t11.*t13;
t34 = t2.*t5.*t12;
t29 = t28-t34;
t30 = sin(t4);
t31 = t18.*t19;
t32 = t14.*t22;
t33 = t31+t32;
t35 = t29.*t30;
t39 = t27.*t33;
t36 = t35-t39;
t37 = t14.*t18;
t41 = t19.*t22;
t38 = t37-t41;
t40 = t26.*t36;
t42 = t23.*t38;
t43 = t40+t42;
t44 = t27.*t29;
t45 = t30.*t33;
t46 = t44+t45;
t47 = t23.*t36;
t49 = t26.*t38;
t48 = t47-t49;
t50 = t2.*t7;
t51 = t6.*t9.*t10;
t52 = t50+t51;
t53 = t5.*t52;
t73 = t6.*t12.*t13;
t54 = t53-t73;
t55 = t2.*t10;
t75 = t6.*t7.*t9;
t56 = t55-t75;
t57 = t10.*t12.*t13.*t24.*8.0;
t58 = t7.*t12.*t14.*t25.*8.0;
t59 = t7.*t12.*t14.*t23.*1.7e1;
t60 = t5.*t7.*t12.*t14.*t23.*1.5e1;
t61 = t10.*t12.*t13.*t23.*t24.*8.0;
t62 = t7.*t12.*t14.*t23.*t25.*8.0;
t63 = t7.*t12.*t13.*t25.*t26.*1.5e1;
t64 = t10.*t12.*t14.*t24.*t26.*1.5e1;
t65 = t7.*t12.*t19.*t24.*t26.*1.7e1;
t66 = t9.*t13.*t14.*t24.*t26.*1.7e1;
t67 = t5.*t10.*t12.*t14.*t24.*t26.*1.7e1;
t68 = t5.*t7.*t12.*t19.*t24.*t26.*1.5e1;
t185 = t5.*t9.*t24.*8.0;
t186 = t9.*t13.*t19.*t25.*8.0;
t187 = t10.*t12.*t19.*t23.*1.5e1;
t188 = t9.*t13.*t19.*t23.*1.7e1;
t189 = t5.*t9.*t23.*t24.*8.0;
t190 = t5.*t10.*t12.*t19.*t25.*8.0;
t191 = t5.*t10.*t12.*t19.*t23.*1.7e1;
t192 = t9.*t13.*t19.*t23.*t25.*8.0;
t193 = t5.*t10.*t12.*t19.*t23.*t25.*8.0;
t69 = t57+t58+t59+t60+t61+t62+t63+t64+t65+t66+t67+t68-t185-t186-t187-t188-t189-t190-t191-t192-t193;
t70 = t13.*t52;
t71 = t5.*t6.*t12;
t72 = t70+t71;
t74 = t19.*t54;
t76 = t14.*t56;
t77 = t74+t76;
t78 = t7.*t12.*t19.*8.0;
t79 = t9.*t13.*t14.*8.0;
t80 = t5.*t10.*t12.*t14.*8.0;
t81 = t10.*t12.*t14.*t25.*1.5e1;
t82 = t7.*t12.*t19.*t25.*1.7e1;
t83 = t9.*t13.*t14.*t25.*1.7e1;
t84 = t7.*t12.*t19.*t23.*8.0;
t85 = t9.*t13.*t14.*t23.*8.0;
t86 = t5.*t10.*t12.*t14.*t25.*1.7e1;
t87 = t5.*t7.*t12.*t19.*t25.*1.5e1;
t88 = t5.*t10.*t12.*t14.*t23.*8.0;
t89 = t10.*t12.*t13.*t25.*t26.*8.0;
t90 = t9.*t13.*t19.*t24.*t26.*8.0;
t91 = t5.*t10.*t12.*t19.*t24.*t26.*8.0;
t210 = t5.*t9.*t25.*t26.*8.0;
t211 = t7.*t12.*t13.*t24.*1.5e1;
t212 = t7.*t12.*t14.*t24.*t26.*8.0;
t92 = t78+t79+t80+t81+t82+t83+t84+t85+t86+t87+t88+t89+t90+t91-t210-t211-t212;
t93 = t30.*t72;
t112 = t27.*t77;
t94 = t93-t112;
t95 = t14.*t54;
t110 = t19.*t56;
t96 = t95-t110;
t97 = t10.*t12.*t19.*t26.*1.5e1;
t98 = t9.*t13.*t19.*t26.*1.7e1;
t99 = t5.*t9.*t24.*t26.*8.0;
t100 = t5.*t10.*t12.*t19.*t26.*1.7e1;
t101 = t9.*t13.*t19.*t25.*t26.*8.0;
t102 = t7.*t12.*t13.*t23.*t25.*1.5e1;
t103 = t10.*t12.*t14.*t23.*t24.*1.5e1;
t104 = t7.*t12.*t19.*t23.*t24.*1.7e1;
t105 = t9.*t13.*t14.*t23.*t24.*1.7e1;
t106 = t5.*t10.*t12.*t19.*t25.*t26.*8.0;
t107 = t5.*t10.*t12.*t14.*t23.*t24.*1.7e1;
t108 = t5.*t7.*t12.*t19.*t23.*t24.*1.5e1;
t204 = t7.*t12.*t14.*t26.*1.7e1;
t205 = t5.*t7.*t12.*t14.*t26.*1.5e1;
t206 = t10.*t12.*t13.*t24.*t26.*8.0;
t207 = t7.*t12.*t14.*t25.*t26.*8.0;
t109 = t97+t98+t99+t100+t101+t102+t103+t104+t105+t106+t107+t108-t204-t205-t206-t207;
t111 = t23.*t96;
t113 = t26.*t94;
t114 = t111+t113;
t115 = t10.*t14.*t25.*8.0;
t116 = t10.*t14.*t23.*1.7e1;
t117 = t7.*t19.*t23.*1.5e1;
t118 = t5.*t7.*t19.*t25.*8.0;
t119 = t5.*t10.*t14.*t23.*1.5e1;
t120 = t5.*t7.*t19.*t23.*1.7e1;
t121 = t10.*t14.*t23.*t25.*8.0;
t122 = t10.*t13.*t25.*t26.*1.5e1;
t123 = t10.*t19.*t24.*t26.*1.7e1;
t124 = t5.*t7.*t19.*t23.*t25.*8.0;
t125 = t5.*t10.*t19.*t24.*t26.*1.5e1;
t215 = t7.*t13.*t24.*8.0;
t216 = t7.*t13.*t23.*t24.*8.0;
t217 = t7.*t14.*t24.*t26.*1.5e1;
t218 = t5.*t7.*t14.*t24.*t26.*1.7e1;
t126 = t115+t116+t117+t118+t119+t120+t121+t122+t123+t124+t125-t215-t216-t217-t218;
t127 = t27.*t72;
t128 = t30.*t77;
t129 = t127+t128;
t130 = t5.*t7.*t14.*8.0;
t131 = t10.*t13.*t24.*1.5e1;
t132 = t7.*t14.*t25.*1.5e1;
t133 = t5.*t7.*t14.*t25.*1.7e1;
t134 = t5.*t7.*t14.*t23.*8.0;
t135 = t7.*t13.*t25.*t26.*8.0;
t136 = t10.*t14.*t24.*t26.*8.0;
t137 = t5.*t7.*t19.*t24.*t26.*8.0;
t225 = t10.*t19.*8.0;
t226 = t10.*t19.*t25.*1.7e1;
t227 = t10.*t19.*t23.*8.0;
t228 = t5.*t10.*t19.*t25.*1.5e1;
t138 = t130+t131+t132+t133+t134+t135+t136+t137-t225-t226-t227-t228;
t139 = t23.*t94;
t156 = t26.*t96;
t140 = t139-t156;
t141 = t10.*t14.*t26.*1.7e1;
t142 = t7.*t19.*t26.*1.5e1;
t143 = t5.*t10.*t14.*t26.*1.5e1;
t144 = t5.*t7.*t19.*t26.*1.7e1;
t145 = t10.*t14.*t25.*t26.*8.0;
t146 = t7.*t14.*t23.*t24.*1.5e1;
t147 = t5.*t7.*t19.*t25.*t26.*8.0;
t148 = t5.*t7.*t14.*t23.*t24.*1.7e1;
t232 = t10.*t13.*t23.*t25.*1.5e1;
t233 = t10.*t19.*t23.*t24.*1.7e1;
t234 = t7.*t13.*t24.*t26.*8.0;
t235 = t5.*t10.*t19.*t23.*t24.*1.5e1;
t149 = t141+t142+t143+t144+t145+t146+t147+t148-t232-t233-t234-t235;
t150 = t5.*t24.*8.0;
t151 = t13.*t19.*t25.*8.0;
t152 = t13.*t19.*t23.*1.7e1;
t153 = t5.*t23.*t24.*8.0;
t154 = t13.*t19.*t23.*t25.*8.0;
t238 = t13.*t14.*t24.*t26.*1.7e1;
t155 = t150+t151+t152+t153+t154-t238;
t157 = t13.*t19.*t26.*1.7e1;
t158 = t5.*t24.*t26.*8.0;
t159 = t13.*t19.*t25.*t26.*8.0;
t160 = t13.*t14.*t23.*t24.*1.7e1;
t161 = t157+t158+t159+t160;
t162 = t13.*t14.*8.0;
t163 = t13.*t14.*t25.*1.7e1;
t164 = t13.*t14.*t23.*8.0;
t165 = t13.*t19.*t24.*t26.*8.0;
t236 = t5.*t25.*t26.*8.0;
t166 = t162+t163+t164+t165-t236;
t167 = t14.*t26.*1.7e1;
t168 = t14.*t25.*t26.*8.0;
t239 = t19.*t23.*t24.*1.7e1;
t169 = t167+t168-t239;
t170 = t14.*t25.*8.0;
t171 = t14.*t23.*1.7e1;
t172 = t14.*t23.*t25.*8.0;
t173 = t19.*t24.*t26.*1.7e1;
t174 = t170+t171+t172+t173;
t175 = t19.*8.0;
t176 = t19.*t25.*1.7e1;
t177 = t19.*t23.*8.0;
t240 = t14.*t24.*t26.*8.0;
t178 = t175+t176+t177-t240;
t179 = t23+1.0;
t180 = t23.*8.0;
t181 = t180+8.0;
t182 = t9.*t13;
t183 = t5.*t10.*t12;
t184 = t182+t183;
t194 = t14.*t184;
t195 = t7.*t12.*t19;
t196 = t194+t195;
t197 = t19.*t184;
t208 = t7.*t12.*t14;
t198 = t197-t208;
t199 = t27.*t198;
t200 = t5.*t9;
t209 = t10.*t12.*t13;
t201 = t200-t209;
t202 = t30.*t201;
t203 = t199+t202;
t213 = t23.*t196;
t237 = t26.*t203;
t214 = t213-t237;
t219 = t9.*t13.*t19;
t220 = t5.*t10.*t12.*t19;
t221 = -t208+t219+t220;
t222 = t25.*t221;
t223 = t24.*t201;
t224 = t222+t223;
t229 = t26.*t196;
t230 = t23.*t203;
t231 = t229+t230;
t241 = t13.*t23.*t25;
t242 = t5.*t19.*t23.*t24;
t276 = t5.*t14.*t26;
t243 = t241+t242-t276;
t244 = t19.*t26;
t245 = t14.*t23.*t24;
t246 = t244+t245;
t247 = t5.*t14.*t23;
t248 = t13.*t25.*t26;
t249 = t5.*t19.*t24.*t26;
t250 = t247+t248+t249;
t251 = t19.*t23;
t262 = t14.*t24.*t26;
t252 = t251-t262;
t253 = t13.*t14.*t26;
t254 = t5.*t23.*t25;
t274 = t13.*t19.*t23.*t24;
t255 = t253+t254-t274;
t256 = t13.*t14.*t23;
t257 = t13.*t19.*t24.*t26;
t263 = t5.*t25.*t26;
t258 = t256+t257-t263;
t259 = t5.*t24;
t260 = t13.*t19.*t25;
t261 = t259+t260;
t264 = t9.*t258;
t265 = t10.*t250;
t266 = t7.*t252;
t267 = t265+t266;
t268 = t12.*t267;
t269 = t264+t268;
t270 = t10.*t13.*t24;
t271 = t7.*t14.*t25;
t289 = t5.*t10.*t19.*t25;
t272 = t270+t271-t289;
t273 = t9.*t261;
t275 = t9.*t255;
t277 = t7.*t246;
t288 = t10.*t243;
t278 = t12.*(t277-t288);
t279 = t275+t278;
t280 = t7.*t243;
t281 = t10.*t246;
t282 = t280+t281;
t283 = t7.*t250;
t291 = t10.*t252;
t284 = t283-t291;
t285 = t10.*t14.*t25;
t286 = t5.*t7.*t19.*t25;
t290 = t7.*t13.*t24;
t287 = t285+t286-t290;
out1 = reshape([t43.*t69+t46.*t92+t48.*t109,-t69.*t114-t92.*t129-t109.*t140,-t69.*t214-t92.*t224+t109.*t231,-t43.*t269+t48.*t279-t46.*(t273-t12.*t272),t114.*t269-t140.*t279+t129.*(t273-t12.*t272),t214.*t269+t231.*t279+t224.*(t273-t12.*t272),t43.*t126-t46.*t138-t48.*t149,-t114.*t126+t129.*t138+t140.*t149,-t126.*t214+t138.*t224-t149.*t231,t43.*t284+t48.*t282+t46.*t287,-t114.*t284-t129.*t287-t140.*t282,-t214.*t284-t224.*t287+t231.*t282,-t43.*t155+t48.*t161+t46.*t166,t114.*t155-t129.*t166-t140.*t161,t155.*t214-t166.*t224+t161.*t231,-t43.*t258+t48.*t255-t46.*t261,t114.*t258+t129.*t261-t140.*t255,t214.*t258+t224.*t261+t231.*t255,t43.*t174-t48.*t169+t46.*t178,-t114.*t174-t129.*t178+t140.*t169,-t174.*t214-t169.*t231-t178.*t224,t48.*t246-t43.*t252+t14.*t25.*t46,t114.*t252-t140.*t246-t14.*t25.*t129,t214.*t252+t231.*t246-t14.*t25.*t224,t25.*t26.*t46.*-8.0+t24.*t26.*t48.*8.0-t24.*t43.*t179.*8.0,t25.*t26.*t129.*8.0-t24.*t26.*t140.*8.0+t24.*t114.*t179.*8.0,t25.*t26.*t224.*8.0+t24.*t26.*t231.*8.0+t24.*t179.*t214.*8.0,-t24.*t46+t25.*t26.*t43+t23.*t25.*t48,t24.*t129-t25.*t26.*t114-t23.*t25.*t140,t24.*t224-t25.*t26.*t214+t23.*t25.*t231,t46.*t181,-t129.*t181,-t181.*t224,-t23.*t43+t26.*t48,t23.*t114-t26.*t140,t23.*t214+t26.*t231,t23.*t38.*-8.0-t26.*t36.*8.0,t23.*t96.*8.0+t26.*t94.*8.0,t23.*t196.*8.0-t26.*t203.*8.0,-t44-t45,t129,t224],[6, 7]);

== matlab function MobileManipulatorSlave/Simulacion/CONTROL system/Cinematica Inversa1/MATLAB Function2 ==
  data: J input; N output
function N = Null(J)
Jp=pinv(J);
I=eye(length(J));
N=(I-Jp*J)';

== matlab function MobileManipulatorSlave/Simulacion/CONTROL system/Cinematica Inversa1/Metodo Cinematico Inverso/Inversa sin singularidad/Inversa Segura ==
  data: u input; y output
function y = fcn(u)

n=length(u);
invu=zeros(n,1);
for i=1:n
    if(abs(u(i))>0.005)
        invu(i)=1/u(i);
    else
        invu(i)=0;
    end
end

y=diag(invu);
